simulink model "ModeloSyncGen2"  (R2014b)
settings: Solver=ode45  StartTime=0.0  StopTime=10.0  RelTol=1e-3
values from neighbouring files (symbols this model uses):
  J = (1/2)*(H*S)/(ws^2)    (= 7029.15711519)    [CalcSteady1.m]    (also in CalcSteady2.m; Main.m = 3.75; Main2.m = 18500)
  Ld = 7e-3    (= 0.007)    [CalcSteady1.m]    (also in CalcSteady2.m; Main.m; Main2.m; SolverODE.m)
  Lf = 7.384e-3    (= 0.007384)    [CalcSteady1.m]    (also in CalcSteady2.m; Main.m; Main2.m; SolverODE.m)
  Lm = 6.656e-3    (= 0.006656)    [CalcSteady1.m]    (also in CalcSteady2.m; Main.m; Main2.m; SolverODE.m)
  Lq = 5.61e-3    (= 0.00561)    [CalcSteady1.m]    (also in CalcSteady2.m; Main.m; Main2.m; SolverODE.m)
  Rf = 0.985e-3    (= 0.000985)    [CalcSteady1.m]    (also in CalcSteady2.m; Main.m; Main2.m; SolverODE.m)
  Rs = 1.6e-3    (= 0.0016)    [CalcSteady1.m]    (also in CalcSteady2.m; Main.m; Main2.m; SolverODE.m)
libraries: dspinverses x1
settings Model: Creator=Eduardo Montilva  LastModifiedBy=Eduardo Montilva

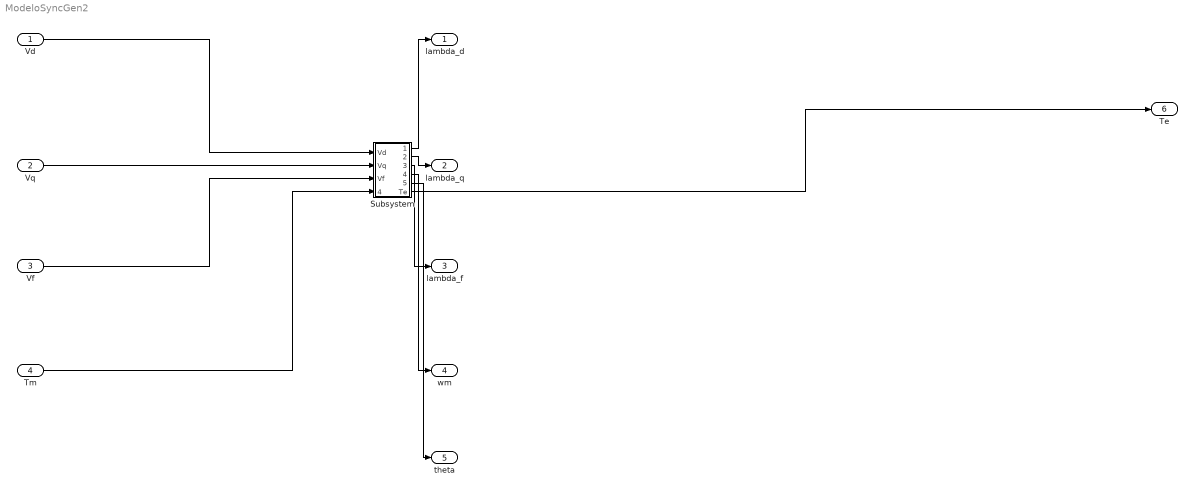
== system ModeloSyncGen2 ==
  Vd : Inport
  Vq : Inport  Port=2
  Vf : Inport  Port=3
  Tm : Inport  Port=4
  Subsystem : Subsystem
  lambda_d : Outport
  lambda_q : Outport  Port=2
  lambda_f : Outport  Port=3
  wm : Outport  Port=4
  theta : Outport  Port=5
  Te : Outport  Port=6
  wires:
  Vd/1 -> Subsystem/1(Vd)
  Vq/1 -> Subsystem/2(Vq)
  Vf/1 -> Subsystem/3(Vf)
  Tm/1 -> Subsystem/4(Tm)
  Subsystem/1(lambda_d) -> lambda_d/1
  Subsystem/2(lambda_q) -> lambda_q/1
  Subsystem/3(lambda_f) -> lambda_f/1
  Subsystem/4(wm) -> wm/1
  Subsystem/5(theta) -> theta/1
  Subsystem/6(Te) -> Te/1

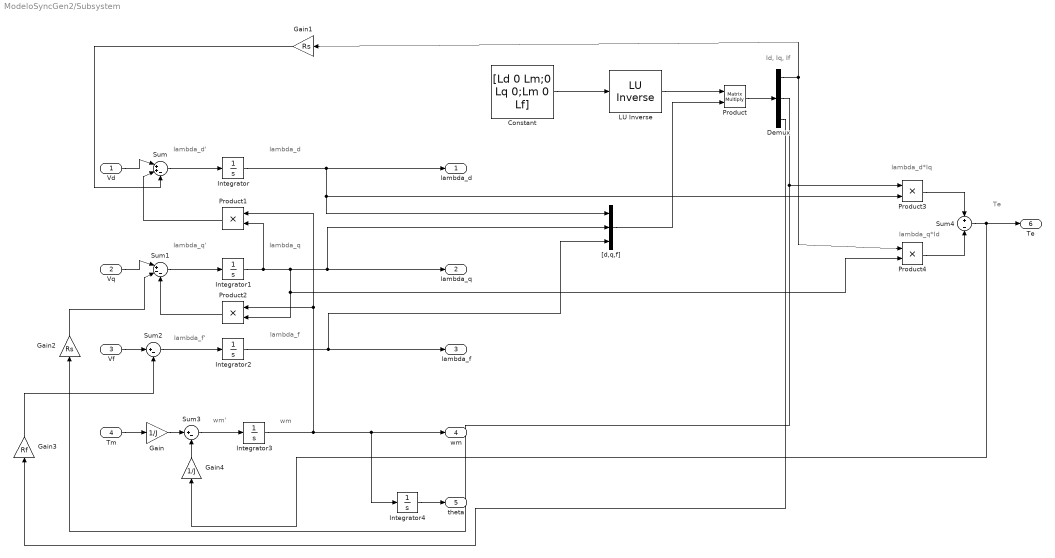
== system ModeloSyncGen2/Subsystem ==
  note: Te
  note: lambda_q*Id
  note: lambda_d*Iq
  note: Id, Iq, If
  note: wm
  note: wm'
  note: lambda_f
  note: lambda_f'
  note: lambda_q
  note: lambda_q'
  note: lambda_d
  note: lambda_d'
  Vd : Inport
  Vq : Inport  Port=2
  Vf : Inport  Port=3
  Tm : Inport  Port=4
  " LU Inverse" : dspinverses/ LU Inverse
  Constant : Constant  Value=[Ld 0 Lm;0 Lq 0;Lm 0 Lf]
  Demux : Demux  Outputs=3
  Gain : Gain  Gain=1/J
  Gain1 : Gain  Gain=Rs
  Gain2 : Gain  Gain=Rs
  Gain3 : Gain  Gain=Rf
  Gain4 : Gain  Gain=1/J
  Integrator{,1..4} (5 alike) : Integrator
  Product : Product  Multiplication=Matrix(*)
  Product{1..4} (4 alike) : Product
  Sum : Sum  Inputs=|++-
  Sum1 : Sum  Inputs=|+--
  Sum2 : Sum  Inputs=|+-
  Sum3 : Sum  Inputs=|+-
  Sum4 : Sum  Inputs=+-
  "[d,q,f]" : Concatenate  NumInputs=3
  lambda_d : Outport
  lambda_q : Outport  Port=2
  lambda_f : Outport  Port=3
  wm : Outport  Port=4
  theta : Outport  Port=5
  Te : Outport  Port=6
  wires:
  Integrator1/1 -> Product1/2, Product4/2, Product2/2, lambda_q/1, "[d,q,f]"/2
  Product1/1 -> Sum/2
  Sum2/1 -> Integrator2/1
  Integrator2/1 -> lambda_f/1, "[d,q,f]"/3
  Integrator/1 -> lambda_d/1, Product3/2, "[d,q,f]"/1
  Vq/1 -> Sum1/1
  Sum1/1 -> Integrator1/1
  Vf/1 -> Sum2/1
  Product/1 -> Demux/1
  Demux/3 -> Gain3/1
  Gain1/1 -> Sum/3
  Demux/2 -> Product3/1, Gain2/1
  Demux/1 -> Gain1/1, Product4/1
  Gain4/1 -> Sum3/2
  Constant/1 -> " LU Inverse"/1
  Sum4/1 -> Te/1, Gain4/1
  Integrator4/1 -> theta/1
  Tm/1 -> Gain/1
  Gain2/1 -> Sum1/2
  Product2/1 -> Sum1/3
  Gain3/1 -> Sum2/2
  Integrator3/1 -> Product2/1, Product1/1, wm/1, Integrator4/1
  Product3/1 -> Sum4/1
  Product4/1 -> Sum4/2
  " LU Inverse"/1 -> Product/1
  "[d,q,f]"/1 -> Product/2
  Sum/1 -> Integrator/1
  Gain/1 -> Sum3/1
  Sum3/1 -> Integrator3/1
  Vd/1 -> Sum/1
